simulink model "HCS_Sim_r9_final"  (R2023a)
settings: Solver=ode4  StartTime=0.0  StopTime=24  FixedStep=5e-3  RelTol=1e-3  EnableMultiTasking=on
libraries: simulink x26, simulink_extras x11, arduinolib x8, spspowerguiLib x1
(part 3 of 5)

== system HCS_Sim_r9_final/untitledPanel2 ==
  Dashboard Scope : DashboardScope  Tag=HiddenForWebPanel  PanelInfo="{\"height\":372,\"left\":38,\"panelId\":\"panelId-fcaf7fae-220a-431c-8918-b7b085aafad7\",\"top\":398,\"type\":\"panelChild\",\"version\":\"2019b\",\"width\":994,\"zIndex\":1500028}"  Ymin=-1.1  Ymax=10  UpdateMode=Scroll
  Display12 : DisplayBlock  Tag=HiddenForWebPanel  PanelInfo="{\"height\":31,\"left\":293,\"panelId\":\"panelId-fcaf7fae-220a-431c-8918-b7b085aafad7\",\"top\":204,\"type\":\"panelChild\",\"version\":\"2019b\",\"width\":94,\"zIndex\":1500020}"  LabelPosition=Hide  Format=bank  Alignment=Left  Transparency=1
  Display15 : DisplayBlock  Tag=HiddenForWebPanel  PanelInfo="{\"height\":26,\"left\":237,\"panelId\":\"panelId-fcaf7fae-220a-431c-8918-b7b085aafad7\",\"top\":282,\"type\":\"panelChild\",\"version\":\"2019b\",\"width\":128,\"zIndex\":1500014}"  LabelPosition=Hide  Format=bank  Alignment=Left  Transparency=1
  Display16 : DisplayBlock  Tag=HiddenForWebPanel  PanelInfo="{\"height\":26,\"left\":237,\"panelId\":\"panelId-fcaf7fae-220a-431c-8918-b7b085aafad7\",\"top\":314,\"type\":\"panelChild\",\"version\":\"2019b\",\"width\":128,\"zIndex\":1500018}"  LabelPosition=Hide  Format=bank  Alignment=Left  Transparency=1
  Display17 : DisplayBlock  Tag=HiddenForWebPanel  PanelInfo="{\"height\":26,\"left\":231,\"panelId\":\"panelId-fcaf7fae-220a-431c-8918-b7b085aafad7\",\"top\":170,\"type\":\"panelChild\",\"version\":\"2019b\",\"width\":128,\"zIndex\":1500024}"  LabelPosition=Hide  Format=bank  Alignment=Left  Transparency=1
  Display18 : DisplayBlock  Tag=HiddenForWebPanel  PanelInfo="{\"height\":26,\"left\":239,\"panelId\":\"panelId-fcaf7fae-220a-431c-8918-b7b085aafad7\",\"top\":247,\"type\":\"panelChild\",\"version\":\"2019b\",\"width\":128,\"zIndex\":1500016}"  LabelPosition=Hide  Format=bank  Alignment=Left  Transparency=1
  Display19 : DisplayBlock  Tag=HiddenForWebPanel  PanelInfo="{\"height\":55,\"left\":592,\"panelId\":\"panelId-fcaf7fae-220a-431c-8918-b7b085aafad7\",\"top\":120,\"type\":\"panelChild\",\"version\":\"2019b\",\"width\":248,\"zIndex\":1500032}"  LabelPosition=Hide  Format=bank  Alignment=Left  Transparency=1  Layout=Fill available space
  Display20 : DisplayBlock  Tag=HiddenForWebPanel  PanelInfo="{\"height\":26,\"left\":231,\"panelId\":\"panelId-fcaf7fae-220a-431c-8918-b7b085aafad7\",\"top\":135,\"type\":\"panelChild\",\"version\":\"2019b\",\"width\":128,\"zIndex\":1500022}"  LabelPosition=Hide  Format=bank  Alignment=Left  Transparency=1
  Display21 : DisplayBlock  Tag=HiddenForWebPanel  PanelInfo="{\"height\":34,\"left\":213,\"panelId\":\"panelId-fcaf7fae-220a-431c-8918-b7b085aafad7\",\"top\":57,\"type\":\"panelChild\",\"version\":\"2019b\",\"width\":113,\"zIndex\":1500026}"  LabelPosition=Hide  Format=bank  Alignment=Left  Transparency=1
  Display22 : DisplayBlock  Tag=HiddenForWebPanel  PanelInfo="{\"height\":55,\"left\":590,\"panelId\":\"panelId-fcaf7fae-220a-431c-8918-b7b085aafad7\",\"top\":181,\"type\":\"panelChild\",\"version\":\"2019b\",\"width\":248,\"zIndex\":1500034}"  LabelPosition=Hide  Alignment=Left  Transparency=1
  Display23 : DisplayBlock  Tag=HiddenForWebPanel  PanelInfo="{\"height\":59,\"left\":591,\"panelId\":\"panelId-fcaf7fae-220a-431c-8918-b7b085aafad7\",\"top\":52,\"type\":\"panelChild\",\"version\":\"2019b\",\"width\":248,\"zIndex\":1500036}"  LabelPosition=Hide  Format=bank  Alignment=Left  Transparency=1  Layout=Fill available space
  panelInfo : PanelWebBlock  Tag=HiddenForWebPanel  PanelInfo="{\"compacted\":false,\"height\":842,\"isActiveTab\":false,\"labels\":{\"label1707239209\":{\"deleted\":false,\"left\":52,\"settings\":{\"backgroundColor\":\"rgba(0, 0, 0, 0)\",\"bold\":true,\"font\":\"Arial\",\"fontColor\":\"black\",\"fontSize\":1.54,\"italicized\":false,\"underlined\":false},\"text\":\"Flywheel Savings: $\",\"top\":207},\"label2728542736\":{\"deleted\":false,\"left\":496,\"settings\":{\"backgroundColor\":\"rgba(0, 0, 0, 0)\",\"bold\":true,\"font\":\"Arial\",\"fontColor\":\"black\",\"fontSize\":1.23,\"italicized\":false,\"underlined\":false},\"text\":\"Time (Hrs)\",\"top\":787},\"label3061890753\":{\"deleted\":false,\"left\":415,\"settings\":{\"backgroundColor\":\"rgba(0, 0, 0, 0)\",\"bold\":false,\"font\":\"Arial\",\"fontColor\":\"black\",\"fontSize\":1.33,\"italicized\":false,\"underlined\":false},\"text\":\"Normal Operation:\",\"top\":69},\"label3961006763\":{\"deleted\":false,\"left\":50,\"settings\":{\"backgroundColor\":\"rgba(0, 0, 0, 0)\",\"bold\":false,\"font\":\"Arial\",\"fontColor\":\"black\",\"fontSize\":1.5,\"italicized\":false,\"underlined\":false},\"text\":\"Flywheel2Grid: $\",\"top\":170},\"label4522966322\":{\"deleted\":false,\"left\":54,\"settings\":{\"backgroundColor\":\"rgba(0, 0, 0, 0)\",\"bold\":true,\"font\":\"Arial\",\"fontColor\":\"#0055ff\",\"fontSize\":1.35,\"italicized\":false,\"underlined\":false},\"text\":\"EV [1] Savings: $\",\"top\":246},\"label4661145740\":{\"deleted\":false,\"left\":411,\"settings\":{\"backgroundColor\":\"rgba(0, 0, 0, 0)\",\"bold\":true,\"font\":\"Arial\",\"fontColor\":\"black\",\"fontSize\":1.64,\"italicized\":false,\"underlined\":false},\"text\":\"Total Cost (per EV, $)\",\"top\":377},\"label5152534318\":{\"deleted\":false,\"left\":44,\"settings\":{\"backgroundColor\":\"rgba(0, 0, 0, 0)\",\"bold\":true,\"font\":\"Lucida Sans\",\"fontColor\":\"black\",\"fontSize\":2.48,\"italicized\":false,\"underlined\":false},\"text\":\"Economics\",\"top\":14},\"label6171120727\":{\"deleted\":false,\"left\":46,\"settings\":{\"backgroundColor\":\"rgba(0, 0, 0, 0)\",\"bold\":false,\"font\":\"Arial\",\"fontColor\":\"black\",\"fontSize\":1.36,\"italicized\":false,\"underlined\":false},\"text\":\"Simulation Time: \",\"top\":59},\"label7378232977\":{\"deleted\":false,\"left\":422,\"settings\":{\"backgroundColor\":\"rgba(0, 0, 0, 0)\",\"bold\":false,\"font\":\"Arial\",\"fontColor\":\"black\",\"fontSize\":1.33,\"italicized\":false,\"underlined\":false},\"text\":\"Smart Operation:\",\"top\":134},\"label7952243197\":{\"deleted\":false,\"left\":49,\"settings\":{\"backgroundColor\":\"rgba(0, 0, 0, 0)\",\"bold\":false,\"font\":\"Arial\",\"fontColor\":\"black\",\"fontSize\":1.5,\"italicized\":false,\"underlined\":false},\"text\":\"Grid2Flywheel: $\",\"top\":137},\"label8040285067\":{\"deleted\":false,\"left\":52,\"settings\":{\"backgroundColor\":\"rgba(0, 0, 0, 0)\",\"bold\":true,\"font\":\"Arial\",\"fontColor\":\"#ff5500\",\"fontSize\":1.36,\"italicized\":false,\"underlined\":false},\"text\":\"EV [2] Savings: $\",\"top\":281},\"label8079460477\":{\"deleted\":false,\"left\":54,\"settings\":{\"backgroundColor\":\"rgba(0, 0, 0, 0)\",\"bold\":true,\"font\":\"Arial\",\"fontColor\":\"#ffcc00\",\"fontSize\":1.36,\"italicized\":false,\"underlined\":false},\"text\":\"EV [3] Savings: $\",\"top\":315},\"label9134032585\":{\"deleted\":false,\"left\":486,\"settings\":{\"backgroundColor\":\"rgba(0, 0, 0, 0)\",\"bold\":false,\"font\":\"Arial\",\"fontColor\":\"black\",\"fontSize\":1.33,\"italicized\":false,\"underlined\":false},\"text\":\"Efficiency:\",\"top\":195}},\"left\":344,\"name\":\"Panel2\",\"panelId\":\"panelId-fcaf7fae-220a-431c-8918-b7b085aafad7\",\"tabIndex\":2,\"tabbedSetId\":\"tabbedSet1419519353\",\"top\":42,\"type\":\"panel\",\"version\":\"2019b\",\"visible\":false,\"width\":1117,\"zIndex\":1500004}"  PanelSnapshot=<binary blob, 120248 chars, not shown>  PanelBackground=data:image/png;base64,iVBORw0KGgoAAAANSUhEUgAAB4AAAAUoCAYAAABNcshsAAAAAXNSR0IArs4c6QAAAARnQU1BAACxjwv8YQUAAAAJcEhZcwAADsQAAA7EAZUrDhsAAJSTSURBVHhe7N11YJ3l2QfgO0ldcZeibXEfw6Zs2IBiG2wwYPg3pAyHYi20WAsTfDDBGboh29hwxnAv7lIotKXUG/nynjxdmvYkOUlOSntyXV14n/tJcnIs++eX+37KamoFAAAAAAAAAAu88nQFAAAAAAAAYAEnAAYAAAAAAAAoEQJgAAAAAAAAgBIhAAYAAAAAAAAoEQJgAAAAAAAAgBIhAAYAAAAAAAAoEQJgAAAAAAAAgBIhAAYAAAAAAAAoEQJgAAAAAAAAgBIhAAYAAAAAAAAoEQJg ...(+50456 chars)
